simulink model "Missile_Aerodynamics"  (R2018a)
settings: Solver=ode4  StartTime=0.0  StopTime=5  FixedStep=Step_Size  RelTol=1e-3  EnableMultiTasking=on
InitFcn:
  | clc ;
  | clear all ;
  | close all ;
  | Missile_Data ;
  | Sim_Parameters ;
undefined symbols (not defined in the file): ALT, D, K_A, K_DC, K_p, K_phi, K_R, Mass, Omega_i, S, SOS_Table, Tbl_ALPHAT, Tbl_CL_ALPHAT, Tbl_CL_DEL_R, Tbl_CL_P, Tbl_CM_0, Tbl_CM_DEL_P, Tbl_CM_PHIT, Tbl_CM_Q, Tbl_CN_DEL_Y, Tbl_CN_PHIT, Tbl_CN_R, Tbl_CX_0, Tbl_CX_ALPHAT, Tbl_CX_DEL_EFF, Tbl_CY_DEL_Y, Tbl_CY_PHIT, Tbl_CZ_0, Tbl_CZ_DEL_P, Tbl_CZ_PHIT, Tbl_MACH, UNIT_GRAV, Wn_Act, XCG, XREF, Zeta_Act
libraries: simulink_extras x8, aerolibtransform2 x4, aerolibconvert2 x3, aerolibasang x3, UAS_Model_library x2, shared6dof x1
settings Model: Creator=e803534  LastModifiedBy=s293701
settings OptimizationCC: LifeSpan=inf
settings DebuggingCC: UnconnectedInputMsg=none  UnconnectedOutputMsg=none  UnconnectedLineMsg=none  LibraryContextMissingDiagnostic=warning  SFUnexpectedBacktrackingDiag=warning  SFNoUnconditionalDefaultTransitionDiag=warning
settings CodeAppCC: StateflowObjectComments=on
settings GRTTargetCC: TargetLangStandard=C89/C90 (ANSI)  GeneratePreprocessorConditionals=Disable all
settings ConfigComp: CovMetricSettings=dw  CovHtmlReporting=on  CovSaveCumulativeToWorkspaceVar=on  CovSaveSingleToWorkspaceVar=on  CovExternalEMLEnable=off

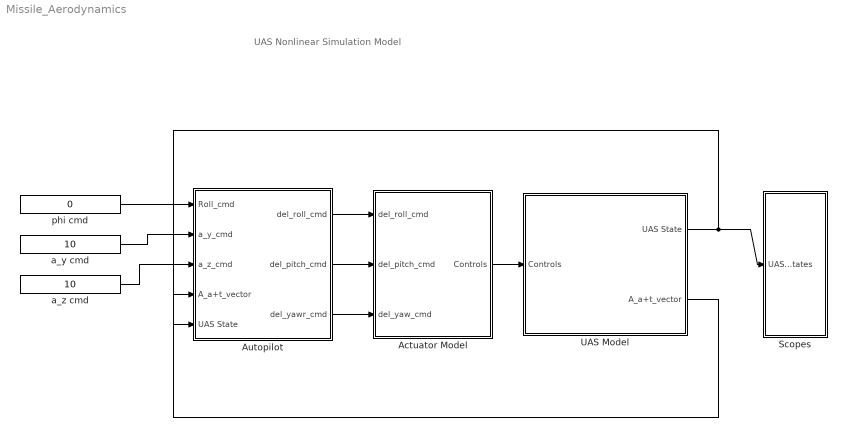
== system Missile_Aerodynamics ==
  note: UAS Nonlinear Simulation Model
  Actuator Model : Subsystem
  "Autopilot " : Subsystem
  Scopes : Subsystem
  UAS Model : Subsystem
  a_y cmd : Constant  Value=10
  a_z cmd : Constant  Value=10
  phi cmd : Constant  Value=0
  wires:
  "Autopilot "/2(del_pitch_cmd) -> Actuator Model/2(del_pitch_cmd)
  "Autopilot "/1(del_roll_cmd) -> Actuator Model/1(del_roll_cmd)
  "Autopilot "/3(del_yawr_cmd) -> Actuator Model/3(del_yaw_cmd)
  UAS Model/1(UAS State) -> "Autopilot "/5(UAS State), Scopes/1(UAS States)
  a_z cmd/1 -> "Autopilot "/3(a_z_cmd)
  phi cmd/1 -> "Autopilot "/1(Roll_cmd)
  a_y cmd/1 -> "Autopilot "/2(a_y_cmd)
  UAS Model/2(A_a+t_vector) -> "Autopilot "/4(A_a+t_vector)
  Actuator Model/1(Controls) -> UAS Model/1(Controls)

== system Missile_Aerodynamics/Actuator Model ==
  note: Actuator Models
  del_roll_cmd : Inport
  del_pitch_cmd : Inport  Port=2
  del_yaw_cmd : Inport  Port=3
  Display : Display
  Display1 : Display
  Display2 : Display
  Mux : Mux  Inputs=3
  Radians to Degrees : simulink_extras/Transformations/Radians to Degrees
  Saturation : Saturate  UpperLimit=10  LowerLimit=-10
  Saturation1 : Saturate  UpperLimit=10  LowerLimit=-10
  Saturation2 : Saturate  UpperLimit=10  LowerLimit=-10
  Scope1 : Scope
  Transfer Fcn : TransferFcn  Numerator=[Wn_Act^2]  Denominator=[1 2*Zeta_Act*Wn_Act Wn_Act^2]
  Transfer Fcn1 : TransferFcn  Numerator=[Wn_Act^2]  Denominator=[1 2*Zeta_Act*Wn_Act Wn_Act^2]
  Transfer Fcn2 : TransferFcn  Numerator=[Wn_Act^2]  Denominator=[1 2*Zeta_Act*Wn_Act Wn_Act^2]
  Controls : Outport
  wires:
  del_roll_cmd/1 -> Transfer Fcn/1
  Mux/1 -> Radians to Degrees/1, Controls/1
  del_yaw_cmd/1 -> Transfer Fcn2/1
  del_pitch_cmd/1 -> Transfer Fcn1/1
  Transfer Fcn/1 -> Saturation/1, Display/1
  Transfer Fcn1/1 -> Display1/1, Saturation1/1
  Transfer Fcn2/1 -> Saturation2/1, Display2/1
  Saturation/1 -> Mux/1
  Saturation2/1 -> Mux/3
  Saturation1/1 -> Mux/2
  Radians to Degrees/1 -> Scope1/1

== system Missile_Aerodynamics/Autopilot  ==
  note: Autopilot
  Roll_cmd : Inport
  a_y_cmd : Inport  Port=2
  a_z_cmd : Inport  Port=3
  A_a+t_vector : Inport  Port=4
  UAS State : Inport  Port=5
  Mux : Mux  Inputs=3
  Pitch Control : Subsystem  AncestorBlock=UAS_Model_library/Autopilot/Pitch Control
  Roll Control : Subsystem  AncestorBlock=UAS_Model_library/Autopilot/Roll Control
  Scope : Scope
  "Yaw Control " : Subsystem  AncestorBlock=UAS_Model_library/Autopilot/Yaw SAS
  del_roll_cmd : Outport
  del_pitch_cmd : Outport  Port=2
  del_yawr_cmd : Outport  Port=3
  wires:
  UAS State/1 -> Pitch Control/2(UAS_State), Roll Control/2(UAS_State), "Yaw Control "/1(UAS_State)
  a_z_cmd/1 -> Pitch Control/1(a_z_cmd)
  Pitch Control/1(del_p_cmd) -> Mux/2, del_pitch_cmd/1
  Roll_cmd/1 -> Roll Control/1(Roll_cmd)
  Roll Control/1(del_r_cmd) -> Mux/1, del_roll_cmd/1
  a_y_cmd/1 -> "Yaw Control "/2("a_y_cmd ")
  "Yaw Control "/1(del_r_cmd) -> Mux/3, del_yawr_cmd/1
  A_a+t_vector/1 -> Pitch Control/3(A_a+t_vector), "Yaw Control "/3(A_a+t_vector)
  Mux/1 -> Scope/1

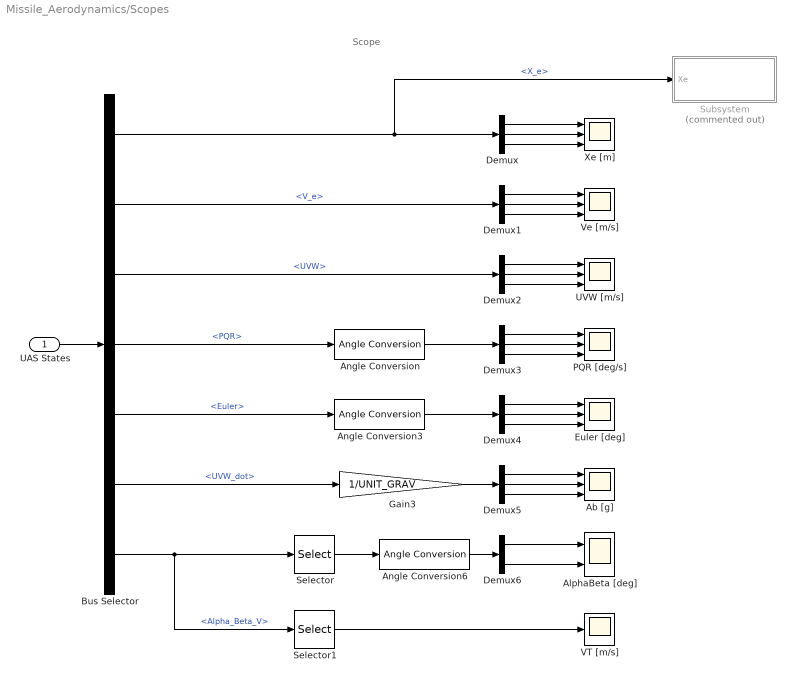
== system Missile_Aerodynamics/Scopes ==
  note: Scope
  UAS States : Inport
  Ab [g] : Scope  NumInputPorts=3
  AlphaBeta [deg] : Scope  NumInputPorts=2
  Angle Conversion : aerolibconvert2/Angle Conversion  IU=rad  OU=deg
  Angle Conversion3 : aerolibconvert2/Angle Conversion  IU=rad  OU=deg
  Angle Conversion6 : aerolibconvert2/Angle Conversion  IU=rad  OU=deg
  Bus Selector : BusSelector  OutputSignals=X_e,V_e,UVW,PQR,Euler,UVW_dot,Alpha_Beta_V
  Demux{,1..5} (6 alike) : Demux  Outputs=3
  Demux6 : Demux  Outputs=2
  Euler [deg] : Scope  NumInputPorts=3
  Gain3 : Gain  Gain=1/UNIT_GRAV
  PQR [deg/s] : Scope  NumInputPorts=3
  Selector : Selector  InputPortWidth=3  IndexOptions=Index vector (dialog)  Indices=[1 2]  OutputSizes=1
  Selector1 : Selector  InputPortWidth=3  IndexOptions=Index vector (dialog)  Indices=[3]  OutputSizes=1
  Subsystem : Subsystem  Commented=on
  UVW [m/s] : Scope  NumInputPorts=3
  VT [m/s] : Scope
  Ve [m/s] : Scope  NumInputPorts=3
  Xe [m] : Scope  NumInputPorts=3
  wires:
  UAS States/1 -> Bus Selector/1
  Bus Selector/1 -> Subsystem/1(Xe), Demux/1  "<X_e>"
  Bus Selector/2 -> Demux1/1  "<V_e>"
  Bus Selector/3 -> Demux2/1  "<UVW>"
  Bus Selector/4 -> Angle Conversion/1  "<PQR>"
  Bus Selector/5 -> Angle Conversion3/1  "<Euler>"
  Bus Selector/6 -> Gain3/1  "<UVW_dot>"
  Angle Conversion3/1 -> Demux4/1
  Angle Conversion/1 -> Demux3/1
  Selector1/1 -> VT [m/s]/1
  Gain3/1 -> Demux5/1
  Demux/1 -> Xe [m]/1
  Demux/2 -> Xe [m]/2
  Demux/3 -> Xe [m]/3
  Demux1/1 -> Ve [m/s]/1
  Demux1/2 -> Ve [m/s]/2
  Demux1/3 -> Ve [m/s]/3
  Demux2/1 -> UVW [m/s]/1
  Demux2/2 -> UVW [m/s]/2
  Demux2/3 -> UVW [m/s]/3
  Demux3/1 -> PQR [deg/s]/1
  Demux3/2 -> PQR [deg/s]/2
  Demux3/3 -> PQR [deg/s]/3
  Demux4/1 -> Euler [deg]/1
  Demux4/2 -> Euler [deg]/2
  Demux4/3 -> Euler [deg]/3
  Demux5/1 -> Ab [g]/1
  Demux5/2 -> Ab [g]/2
  Demux5/3 -> Ab [g]/3
  Demux6/2 -> AlphaBeta [deg]/2
  Demux6/1 -> AlphaBeta [deg]/1
  Angle Conversion6/1 -> Demux6/1
  Bus Selector/7 -> Selector1/1, Selector/1  "<Alpha_Beta_V>"
  Selector/1 -> Angle Conversion6/1

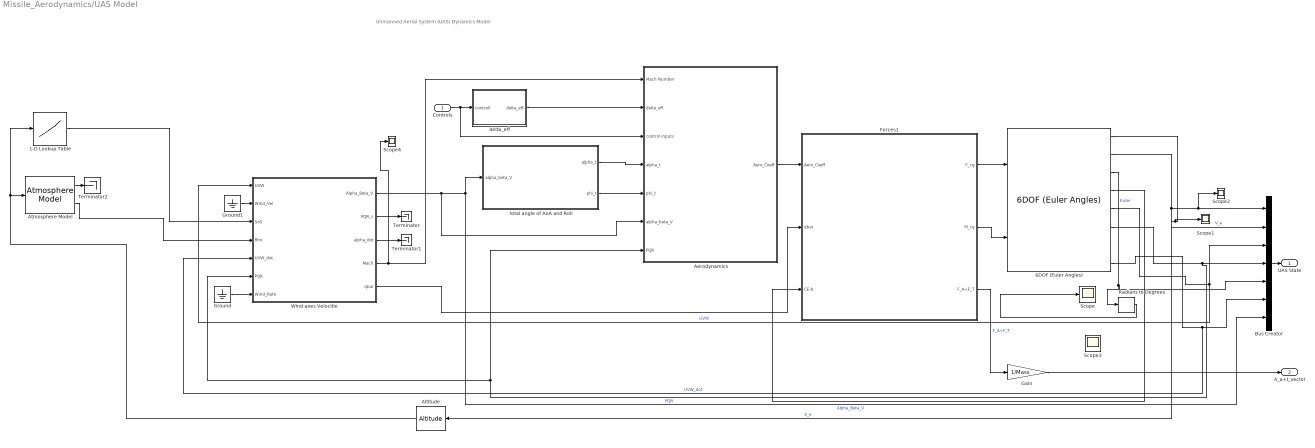
== system Missile_Aerodynamics/UAS Model ==
  note: Unmanned Aerial System (UAS) Dynamics Model
  Controls : Inport
  1-D Lookup Table : Lookup_n-D  NumberOfTableDimensions=1  BreakpointsForDimension1=ALT  Table=SOS_Table  InternalRulePriority=Speed  RndMeth=Simplest  InputSameDT=on
  6DOF (Euler Angles) : shared6dof/6DOF (Euler Angles)  units=Metric (MKS)  mtype=Fixed  rep=Euler Angles  xme_0=Init_Pos  Vm_0=Init_Vel  eul_0=Init_Euler  pm_0=Init_Rate  mass_0=Mass  mass_e=0.5  mass_f=2.0  inertia=I_TENSOR  inertia_e=eye(3)  inertia_f=2*eye(3)  k_quat=1.0  vre_flag=on  abi_flag=off  aMode=0
      settings: SourceProductBaseCode=AE
  Aerodynamics : Subsystem
  Altitude : UAS_Model_library/Equations of Motion/Altitude
  Atmosphere Model : UAS_Model_library/Envrionment/Atmosphere Model
  Bus Creator : BusCreator  Inputs=7
  Forces1 : Subsystem
  Gain : Gain  Gain=1/Mass
  Ground : Ground
  Ground1 : Ground
  Radians to Degrees : simulink_extras/Transformations/Radians to Degrees
  Scope{,1..4} (5 alike) : Scope
  Terminator : Terminator
  Terminator1 : Terminator
  Terminator2 : Terminator
  Wind-axes Velocitie : Subsystem  AncestorBlock=UAS_Model_library/External Forces/Aerodynamics/Wind-axes Velocitie
  delta_eff : Subsystem
  total angle of AoA and Roll : Subsystem
  UAS State : Outport
  A_a+t_vector : Outport  Port=2
  wires:
  Wind-axes Velocitie/1(Alpha_Beta_V) -> Aerodynamics/6(alpha_beta_V), total angle of AoA and Roll/1(alpha_beta_V), Bus Creator/7  "Alpha_Beta_V"
  total angle of AoA and Roll/2(phi_t) -> Aerodynamics/5(phi_t)
  delta_eff/1(delta_eff) -> Aerodynamics/2(delta_eff)
  Atmosphere Model/2 -> Wind-axes Velocitie/4(Rho)
  6DOF (Euler Angles)/8 -> Bus Creator/6, Wind-axes Velocitie/5(UVW_dot)  "UVW_dot"
  total angle of AoA and Roll/1(alpha_t) -> Aerodynamics/4(alpha_t)
  Wind-axes Velocitie/4(Mach) -> Scope4/1, Aerodynamics/1(Mach Number)
  6DOF (Euler Angles)/5 -> Wind-axes Velocitie/1(UVW), Bus Creator/3  "UVW"
  Ground1/1 -> Wind-axes Velocitie/2(Wind_Vel)
  Forces1/1(F_cg) -> 6DOF (Euler Angles)/1
  Aerodynamics/1(Aero_Coeff) -> Forces1/1(Aero_Coeff)
  Forces1/2(M_cg) -> 6DOF (Euler Angles)/2
  6DOF (Euler Angles)/6 -> Wind-axes Velocitie/6(PQR), Aerodynamics/7(PQR), Bus Creator/4  "PQR"
  Controls/1 -> Aerodynamics/3(control inputs), delta_eff/1(controll)
  Wind-axes Velocitie/5(qbar) -> Forces1/2(qbar)
  Ground/1 -> Wind-axes Velocitie/7(Wind_Rate)
  Bus Creator/1 -> UAS State/1
  6DOF (Euler Angles)/2 -> Altitude/1, Scope2/1, Bus Creator/1  "X_e"
  6DOF (Euler Angles)/1 -> Bus Creator/2, Scope1/1  "V_e"
  6DOF (Euler Angles)/3 -> Radians to Degrees/1, Bus Creator/5  "Euler"
  Forces1/3(F_A+F_T) -> Gain/1  "F_A+F_T"
  Wind-axes Velocitie/2(PQR_s) -> Terminator/1
  Wind-axes Velocitie/3(alpha_dot) -> Terminator1/1
  6DOF (Euler Angles)/4 -> Forces1/3(CE-b)
  Altitude/1 -> 1-D Lookup Table/1, Atmosphere Model/1
  Radians to Degrees/1 -> Scope/1
  Gain/1 -> A_a+t_vector/1
  Atmosphere Model/1 -> Terminator2/1
  1-D Lookup Table/1 -> Wind-axes Velocitie/3(SoS)

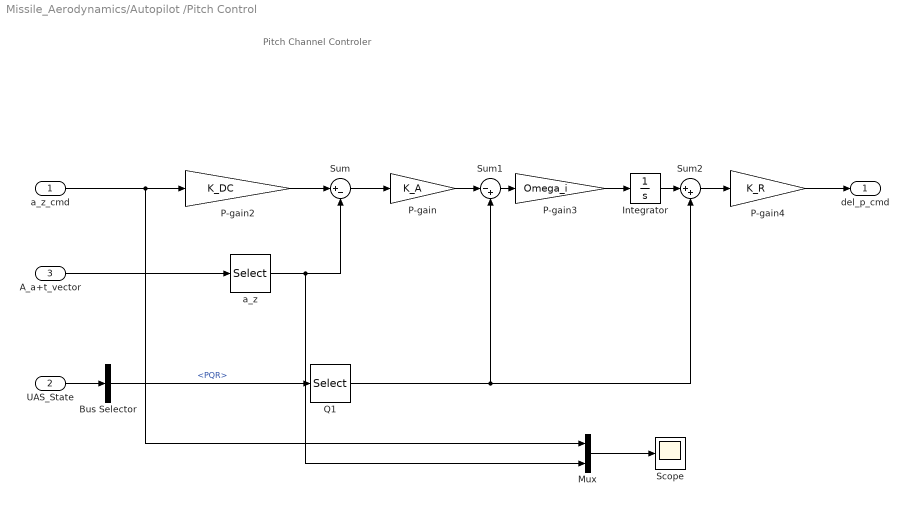
== system Missile_Aerodynamics/Autopilot /Pitch Control ==
  note: Pitch Channel Controler
  a_z_cmd : Inport
  UAS_State : Inport  Port=2
  A_a+t_vector : Inport  Port=3
  Bus Selector : BusSelector  OutputSignals=PQR
  Integrator : Integrator
  Mux : Mux  Inputs=2
  P-gain : Gain  Gain=K_A
  P-gain2 : Gain  Gain=K_DC
  P-gain3 : Gain  Gain=Omega_i
  P-gain4 : Gain  Gain=K_R
  Q1 : Selector  InputPortWidth=3  IndexOptions=Index vector (dialog)  Indices=[2]  OutputSizes=1
  Scope : Scope
  Sum : Sum  Inputs=|+-
  Sum1 : Sum  Inputs=|-+
  Sum2 : Sum  Inputs=|++
  a_z : Selector  InputPortWidth=3  IndexOptions=Index vector (dialog)  Indices=[3]  OutputSizes=1
  del_p_cmd : Outport
  wires:
  UAS_State/1 -> Bus Selector/1
  Bus Selector/1 -> Q1/1  "<PQR>"
  Sum2/1 -> P-gain4/1
  Sum1/1 -> P-gain3/1
  Q1/1 -> Sum2/2, Sum1/2
  P-gain/1 -> Sum1/1
  Sum/1 -> P-gain/1
  a_z_cmd/1 -> Mux/1, P-gain2/1
  P-gain2/1 -> Sum/1
  P-gain3/1 -> Integrator/1
  Integrator/1 -> Sum2/1
  P-gain4/1 -> del_p_cmd/1
  a_z/1 -> Mux/2, Sum/2
  A_a+t_vector/1 -> a_z/1
  Mux/1 -> Scope/1

== system Missile_Aerodynamics/Autopilot /Roll Control ==
  note: Roll Control
  Roll_cmd : Inport
  UAS_State : Inport  Port=2
  Bus Selector : BusSelector  OutputSignals=Euler,PQR
  P : Selector  InputPortWidth=3  IndexOptions=Index vector (dialog)  Indices=[1]  OutputSizes=1
  P-gain2 : Gain  Gain=K_phi
  P-gain3 : Gain  Gain=K_p
  PHI : Selector  InputPortWidth=3  IndexOptions=Index vector (dialog)  Indices=[1]  OutputSizes=1
  Sum : Sum  Inputs=|+-
  Sum2 : Sum  Inputs=|+-
  del_r_cmd : Outport
  wires:
  Bus Selector/2 -> P/1  "<PQR>"
  Bus Selector/1 -> PHI/1  "<Euler>"
  UAS_State/1 -> Bus Selector/1
  PHI/1 -> Sum/2
  Roll_cmd/1 -> Sum/1
  P-gain2/1 -> Sum2/1
  P/1 -> Sum2/2
  Sum2/1 -> P-gain3/1
  Sum/1 -> P-gain2/1
  P-gain3/1 -> del_r_cmd/1

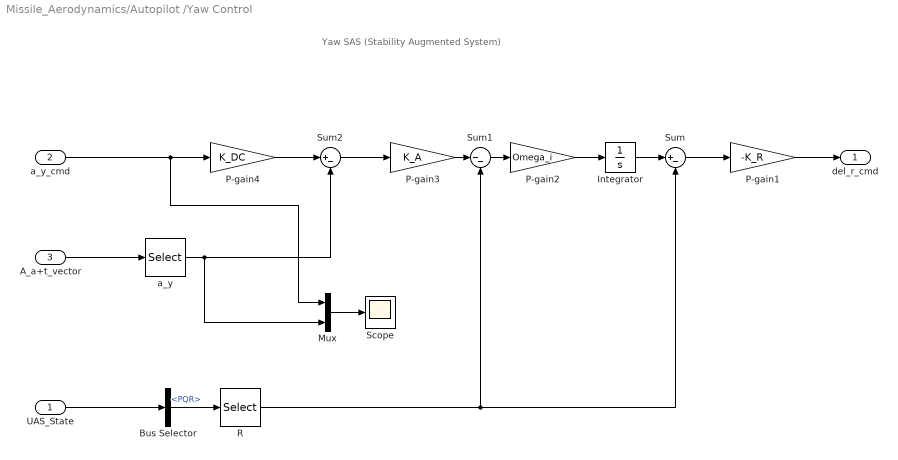
== system Missile_Aerodynamics/Autopilot /Yaw Control  ==
  note: Yaw SAS (Stability Augmented System)
  UAS_State : Inport
  "a_y_cmd " : Inport  Port=2
  A_a+t_vector : Inport  Port=3
  Bus Selector : BusSelector  OutputSignals=PQR
  Integrator : Integrator
  Mux : Mux  Inputs=2
  P-gain1 : Gain  Gain=-K_R
  P-gain2 : Gain  Gain=Omega_i
  P-gain3 : Gain  Gain=K_A
  P-gain4 : Gain  Gain=K_DC
  R : Selector  InputPortWidth=3  IndexOptions=Index vector (dialog)  Indices=[3]  OutputSizes=1
  Scope : Scope
  Sum : Sum  Inputs=|+-
  Sum1 : Sum  Inputs=|--
  Sum2 : Sum  Inputs=|+-
  a_y : Selector  InputPortWidth=3  IndexOptions=Index vector (dialog)  Indices=[2]  OutputSizes=1
  del_r_cmd : Outport
  wires:
  P-gain1/1 -> del_r_cmd/1
  P-gain2/1 -> Integrator/1
  Sum/1 -> P-gain1/1
  Integrator/1 -> Sum/1
  Sum1/1 -> P-gain2/1
  P-gain3/1 -> Sum1/1
  Sum2/1 -> P-gain3/1
  Bus Selector/1 -> R/1  "<PQR>"
  P-gain4/1 -> Sum2/1
  R/1 -> Sum1/2, Sum/2
  "a_y_cmd "/1 -> Mux/1, P-gain4/1
  UAS_State/1 -> Bus Selector/1
  A_a+t_vector/1 -> a_y/1
  a_y/1 -> Mux/2, Sum2/2
  Mux/1 -> Scope/1

== system Missile_Aerodynamics/Scopes/Subsystem ==
  Xe : Inport
  Constant : Constant
  Constant1 : Constant  Value=0
  Selector : Selector  InputPortWidth=3  IndexOptions=Index vector (dialog)  Indices=[3]  OutputSizes=1
  Stop Simulation : Stop
  Switch : Switch  Criteria=u2 > Threshold
  wires:
  Xe/1 -> Selector/1
  Selector/1 -> Switch/2
  Constant/1 -> Switch/1
  Constant1/1 -> Switch/3
  Switch/1 -> Stop Simulation/1

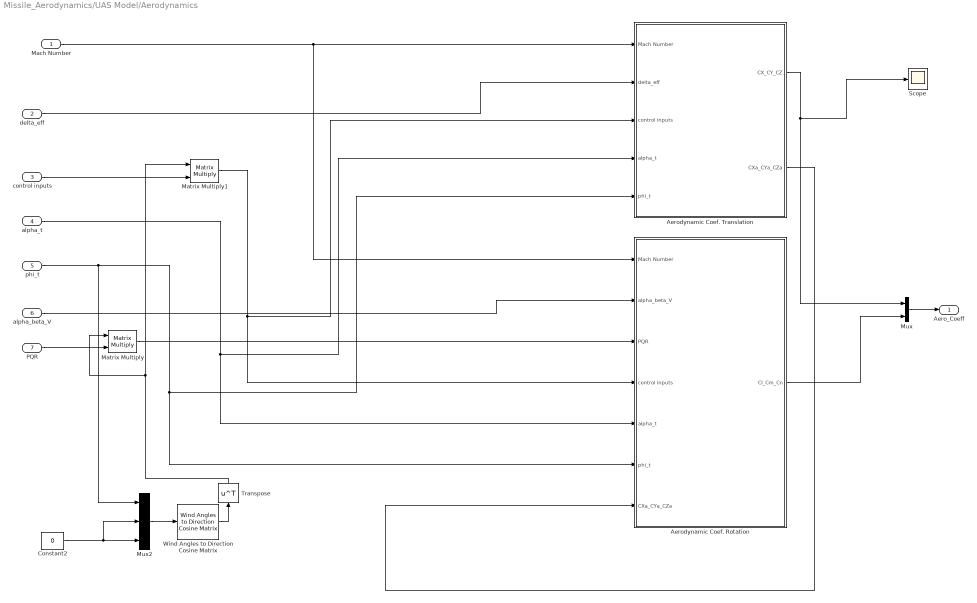
== system Missile_Aerodynamics/UAS Model/Aerodynamics ==
  Mach Number : Inport
  delta_eff : Inport  Port=2
  control inputs : Inport  Port=3
  alpha_t : Inport  Port=4
  phi_t : Inport  Port=5
  alpha_beta_V : Inport  Port=6
  PQR : Inport  Port=7
  Aerodynamic Coef. Rotation : Subsystem
  Aerodynamic Coef. Translation : Subsystem
  Constant2 : Constant  Value=0
  Matrix Multiply : Product  Multiplication=Matrix(*)
  Matrix Multiply1 : Product  Multiplication=Matrix(*)
  Mux : Mux  Inputs=2
  Mux2 : Mux  Inputs=3
  Scope : Scope
  Transpose : Math  Operator=transpose  SaturateOnIntegerOverflow=on
  Wind Angles to Direction Cosine Matrix : aerolibtransform2/Wind Angles to  Direction Cosine Matrix
      settings: SourceProductName=Aerospace Blockset  SourceProductBaseCode=AE
  Aero_Coeff : Outport
  wires:
  Aerodynamic Coef. Translation/2(CXa_CYa_CZa) -> Aerodynamic Coef. Rotation/7(CXa_CYa_CZa)
  Mach Number/1 -> Aerodynamic Coef. Rotation/1(Mach Number), Aerodynamic Coef. Translation/1(Mach Number)
  delta_eff/1 -> Aerodynamic Coef. Translation/2(delta_eff)
  Matrix Multiply1/1 -> Aerodynamic Coef. Rotation/4(control inputs), Aerodynamic Coef. Translation/3(control inputs)
  alpha_beta_V/1 -> Aerodynamic Coef. Rotation/2(alpha_beta_V)
  Matrix Multiply/1 -> Aerodynamic Coef. Rotation/3(PQR)
  Aerodynamic Coef. Translation/1(CX_CY_CZ) -> Scope/1, Mux/1
  Aerodynamic Coef. Rotation/1(Cl_Cm_Cn) -> Mux/2
  Mux/1 -> Aero_Coeff/1
  alpha_t/1 -> Aerodynamic Coef. Rotation/5(alpha_t), Aerodynamic Coef. Translation/4(alpha_t)
  phi_t/1 -> Mux2/1, Aerodynamic Coef. Translation/5(phi_t), Aerodynamic Coef. Rotation/6(phi_t)
  Mux2/1 -> Wind Angles to Direction Cosine Matrix/1
  Constant2/1 -> Mux2/2, Mux2/3
  control inputs/1 -> Matrix Multiply1/2
  Wind Angles to Direction Cosine Matrix/1 -> Transpose/1
  PQR/1 -> Matrix Multiply/2
  Transpose/1 -> Matrix Multiply/1, Matrix Multiply1/1

== system Missile_Aerodynamics/UAS Model/Forces1 ==
  Aero_Coeff : Inport
  qbar : Inport  Port=2
  CE-b : Inport  Port=3
  Aerodynamic Force & Moment : Subsystem  AncestorBlock=UAS_Model_library/External Forces/Aerodynamics/Aerodynamic Force & Moment
  Propulsive Force & Moment : Subsystem  AncestorBlock=UAS_Model_library/External Forces/Propulsive/Propulsive Force & Moment
  Sum of Aerodynamic and Propulsion Forces : Sum
  Total Force & Moment : Subsystem  AncestorBlock=UAS_Model_library/External Forces/Total Force & Moment
  F_cg : Outport
  M_cg : Outport  Port=2
  F_A+F_T : Outport  Port=3
  wires:
  Total Force & Moment/2(M_cg) -> M_cg/1
  Aerodynamic Force & Moment/2(M_aero) -> Total Force & Moment/2(M_aero)
  Propulsive Force & Moment/2(M_prop) -> Total Force & Moment/4(M_prop)
  Total Force & Moment/1(F_cg) -> F_cg/1
  Aerodynamic Force & Moment/1(F_aero) -> Sum of Aerodynamic and Propulsion Forces/1, Total Force & Moment/1(F_aero)
  Propulsive Force & Moment/1(F_prop) -> Sum of Aerodynamic and Propulsion Forces/2, Total Force & Moment/3(F_prop)
  qbar/1 -> Aerodynamic Force & Moment/2(qbar)
  Aero_Coeff/1 -> Aerodynamic Force & Moment/1(Aero_Coeff)
  Sum of Aerodynamic and Propulsion Forces/1 -> F_A+F_T/1
  CE-b/1 -> Total Force & Moment/5("cE-B ")

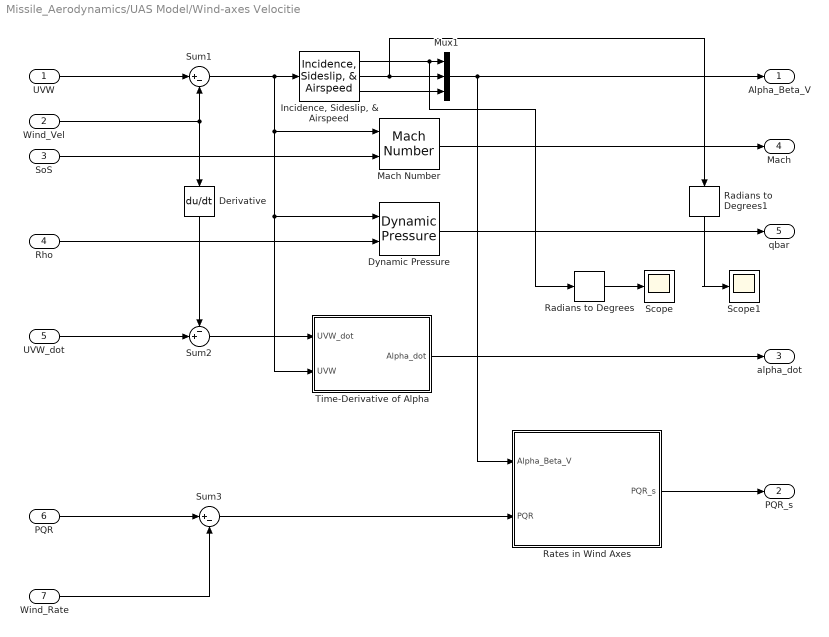
== system Missile_Aerodynamics/UAS Model/Wind-axes Velocitie ==
  UVW : Inport
  Wind_Vel : Inport  Port=2
  SoS : Inport  Port=3
  Rho : Inport  Port=4
  UVW_dot : Inport  Port=5
  PQR : Inport  Port=6
  Wind_Rate : Inport  Port=7
  Derivative : Derivative
  Dynamic Pressure : aerolibasang/Dynamic Pressure
  "Incidence, Sideslip, & Airspeed" : aerolibasang/Incidence, Sideslip, & Airspeed
      settings: SourceProductName=Aerospace Blockset
  Mach Number : aerolibasang/Mach Number
      settings: SourceProductName=Aerospace Blockset  SourceProductBaseCode=AE
  Mux1 : Mux  Inputs=3
  Radians to Degrees : simulink_extras/Transformations/Radians to Degrees
  Radians to Degrees1 : simulink_extras/Transformations/Radians to Degrees
  Rates in Wind Axes : Subsystem
  Scope : Scope
  Scope1 : Scope
  Sum1 : Sum  Inputs=|+-  SaturateOnIntegerOverflow=on  InputSameDT=on  OutDataTypeStr=Inherit: Same as first input
  Sum2 : Sum  Inputs=-+|  SaturateOnIntegerOverflow=on  InputSameDT=on  OutDataTypeStr=Inherit: Same as first input
  Sum3 : Sum  Inputs=|+-  SaturateOnIntegerOverflow=on  InputSameDT=on  OutDataTypeStr=Inherit: Same as first input
  Time-Derivative of Alpha : Subsystem
  Alpha_Beta_V : Outport
  PQR_s : Outport  Port=2
  alpha_dot : Outport  Port=3
  Mach : Outport  Port=4
  qbar : Outport  Port=5
  wires:
  Wind_Rate/1 -> Sum3/2
  PQR/1 -> Sum3/1
  Sum3/1 -> Rates in Wind Axes/2(PQR)
  Rates in Wind Axes/1(PQR_s) -> PQR_s/1
  "Incidence, Sideslip, & Airspeed"/3 -> Mux1/3
  "Incidence, Sideslip, & Airspeed"/2 -> Radians to Degrees1/1, Mux1/2
  "Incidence, Sideslip, & Airspeed"/1 -> Radians to Degrees/1, Mux1/1
  Sum1/1 -> "Incidence, Sideslip, & Airspeed"/1, Mach Number/1, Dynamic Pressure/1, Time-Derivative of Alpha/2(UVW)
  Mux1/1 -> Alpha_Beta_V/1, Rates in Wind Axes/1(Alpha_Beta_V)
  UVW/1 -> Sum1/1
  Wind_Vel/1 -> Derivative/1, Sum1/2
  Mach Number/1 -> Mach/1
  SoS/1 -> Mach Number/2
  Rho/1 -> Dynamic Pressure/2
  Dynamic Pressure/1 -> qbar/1
  Time-Derivative of Alpha/1(Alpha_dot) -> alpha_dot/1
  UVW_dot/1 -> Sum2/2
  Sum2/1 -> Time-Derivative of Alpha/1(UVW_dot)
  Derivative/1 -> Sum2/1
  Radians to Degrees/1 -> Scope/1
  Radians to Degrees1/1 -> Scope1/1

== system Missile_Aerodynamics/UAS Model/delta_eff ==
  controll : Inport
  Abs : Abs
  Abs1 : Abs
  Constant : Constant  Value=2
  Divide : Product  Inputs=*/  SaturateOnIntegerOverflow=on  RndMeth=Zero
  Selector : Selector  InputPortWidth=3  IndexOptions=Index vector (dialog)  Indices=[3]  OutputSizes=1
  Selector1 : Selector  InputPortWidth=3  IndexOptions=Index vector (dialog)  Indices=[2]  OutputSizes=1
  Sum : Sum  Inputs=|++
  delta_eff : Outport
  wires:
  Selector1/1 -> Abs1/1
  Sum/1 -> Divide/1
  Constant/1 -> Divide/2
  Divide/1 -> delta_eff/1
  controll/1 -> Selector/1, Selector1/1
  Selector/1 -> Abs/1
  Abs/1 -> Sum/1
  Abs1/1 -> Sum/2

== system Missile_Aerodynamics/UAS Model/total angle of AoA and Roll ==
  alpha_beta_V : Inport
  Asin : Trigonometry  Operator=acos
  Atan2 : Trigonometry  Operator=atan2
  Cos : Trigonometry  Operator=cos
  Cos1 : Trigonometry  Operator=cos
  Multiply : Product
  Selector : Selector  InputPortWidth=3  IndexOptions=Index vector (dialog)  Indices=[1]  OutputSizes=1
  Selector1 : Selector  InputPortWidth=3  IndexOptions=Index vector (dialog)  Indices=[2]  OutputSizes=1
  Sin : Trigonometry
  Tan : Trigonometry  Operator=tan
  alpha_t : Outport
  phi_t : Outport  Port=2
  wires:
  Sin/1 -> Atan2/2
  Tan/1 -> Atan2/1
  Selector/1 -> Sin/1, Cos/1
  Selector1/1 -> Tan/1, Cos1/1
  Cos1/1 -> Multiply/2
  Multiply/1 -> Asin/1
  Cos/1 -> Multiply/1
  Atan2/1 -> phi_t/1
  Asin/1 -> alpha_t/1
  alpha_beta_V/1 -> Selector1/1, Selector/1

== system Missile_Aerodynamics/UAS Model/Aerodynamics/Aerodynamic Coef. Rotation ==
  Mach Number : Inport
  alpha_beta_V : Inport  Port=2
  PQR : Inport  Port=3
  control inputs : Inport  Port=4
  alpha_t : Inport  Port=5
  phi_t : Inport  Port=6
  CXa_CYa_CZa : Inport  Port=7
  Constant2 : Constant  Value=0
  Display1 : Display
  Matrix Multiply : Product  Multiplication=Matrix(*)
  Mux : Mux  Inputs=3
  Mux2 : Mux  Inputs=3
  Subsystem Aero. Coef. Rotation : Subsystem
  Wind Angles to Direction Cosine Matrix : aerolibtransform2/Wind Angles to  Direction Cosine Matrix
      settings: SourceProductName=Aerospace Blockset  SourceProductBaseCode=AE
  Cl_Cm_Cn : Outport
  wires:
  Mux/1 -> Matrix Multiply/2
  Matrix Multiply/1 -> Cl_Cm_Cn/1
  Mach Number/1 -> Subsystem Aero. Coef. Rotation/1(Mach Number)
  alpha_beta_V/1 -> Subsystem Aero. Coef. Rotation/4(alpha_beta_V)
  PQR/1 -> Subsystem Aero. Coef. Rotation/5(PQR)
  control inputs/1 -> Subsystem Aero. Coef. Rotation/6(control)
  alpha_t/1 -> Subsystem Aero. Coef. Rotation/2(alpha_t)
  phi_t/1 -> Mux2/1, Subsystem Aero. Coef. Rotation/3(phi_t)
  CXa_CYa_CZa/1 -> Subsystem Aero. Coef. Rotation/7(C_X_C_Y_CZ)
  Mux2/1 -> Wind Angles to Direction Cosine Matrix/1
  Constant2/1 -> Mux2/2, Mux2/3
  Wind Angles to Direction Cosine Matrix/1 -> Matrix Multiply/1
  Subsystem Aero. Coef. Rotation/1(C_L_A) -> Mux/1
  Subsystem Aero. Coef. Rotation/2(C_M_A) -> Display1/1, Mux/2
  Subsystem Aero. Coef. Rotation/3(C_N_A) -> Mux/3

== system Missile_Aerodynamics/UAS Model/Aerodynamics/Aerodynamic Coef. Translation ==
  Mach Number : Inport
  delta_eff : Inport  Port=2
  control inputs : Inport  Port=3
  alpha_t : Inport  Port=4
  phi_t : Inport  Port=5
  Constant2 : Constant  Value=0
  Matrix Multiply : Product  Multiplication=Matrix(*)
  Mux : Mux  Inputs=3
  Mux2 : Mux  Inputs=3
  Scope : Scope
  Subsystem Aero. Coef. Translation : Subsystem
  Transpose : Math  Commented=on  Operator=transpose  SaturateOnIntegerOverflow=on
  Wind Angles to Direction Cosine Matrix : aerolibtransform2/Wind Angles to  Direction Cosine Matrix
      settings: SourceProductName=Aerospace Blockset  SourceProductBaseCode=AE
  CX_CY_CZ : Outport
  CXa_CYa_CZa : Outport  Port=2
  wires:
  Mux/1 -> Matrix Multiply/2, CXa_CYa_CZa/1
  Matrix Multiply/1 -> CX_CY_CZ/1
  Mux2/1 -> Wind Angles to Direction Cosine Matrix/1
  phi_t/1 -> Mux2/1, Subsystem Aero. Coef. Translation/5(phi_t)
  Constant2/1 -> Mux2/2, Mux2/3
  Mach Number/1 -> Subsystem Aero. Coef. Translation/1(Mach number)
  control inputs/1 -> Subsystem Aero. Coef. Translation/4(control)
  alpha_t/1 -> Subsystem Aero. Coef. Translation/2(alpha_t)
  delta_eff/1 -> Subsystem Aero. Coef. Translation/3(delta_eff)
  Subsystem Aero. Coef. Translation/1(C_X_A) -> Scope/1, Mux/1
  Subsystem Aero. Coef. Translation/2(C_Y_A) -> Mux/2
  Subsystem Aero. Coef. Translation/3(C_Z_A) -> Mux/3
  Wind Angles to Direction Cosine Matrix/1 -> Matrix Multiply/1

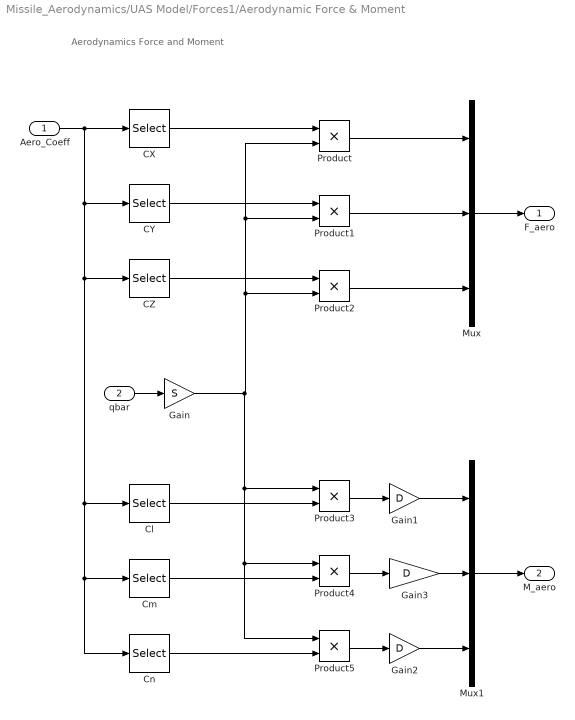
== system Missile_Aerodynamics/UAS Model/Forces1/Aerodynamic Force & Moment ==
  note: Aerodynamics Force and Moment
  Aero_Coeff : Inport
  qbar : Inport  Port=2
  CX : Selector  InputPortWidth=6  IndexOptions=Index vector (dialog)  Indices=[1]  OutputSizes=1
  CY : Selector  InputPortWidth=6  IndexOptions=Index vector (dialog)  Indices=[2]  OutputSizes=1
  CZ : Selector  InputPortWidth=6  IndexOptions=Index vector (dialog)  Indices=[3]  OutputSizes=1
  Cl : Selector  InputPortWidth=6  IndexOptions=Index vector (dialog)  Indices=[4]  OutputSizes=1
  Cm : Selector  InputPortWidth=6  IndexOptions=Index vector (dialog)  Indices=[5]  OutputSizes=1
  Cn : Selector  InputPortWidth=6  IndexOptions=Index vector (dialog)  Indices=[6]  OutputSizes=1
  Gain : Gain  Gain=S
  Gain1 : Gain  Gain=D
  Gain2 : Gain  Gain=D
  Gain3 : Gain  Gain=D
  Mux : Mux  Inputs=3
  Mux1 : Mux  Inputs=3
  Product{,1..5} (6 alike) : Product
  F_aero : Outport
  M_aero : Outport  Port=2
  wires:
  Gain3/1 -> Mux1/2
  Gain2/1 -> Mux1/3
  Gain1/1 -> Mux1/1
  Mux1/1 -> M_aero/1
  Product5/1 -> Gain2/1
  Product4/1 -> Gain3/1
  Product3/1 -> Gain1/1
  Cn/1 -> Product5/2
  Cm/1 -> Product4/2
  Cl/1 -> Product3/2
  Mux/1 -> F_aero/1
  Product2/1 -> Mux/3
  Product1/1 -> Mux/2
  Product/1 -> Mux/1
  CZ/1 -> Product2/1
  CY/1 -> Product1/1
  Gain/1 -> Product/2, Product1/2, Product2/2, Product3/1, Product4/1, Product5/1
  CX/1 -> Product/1
  qbar/1 -> Gain/1
  Aero_Coeff/1 -> CX/1, CY/1, CZ/1, Cm/1, Cn/1, Cl/1

== system Missile_Aerodynamics/UAS Model/Forces1/Propulsive Force & Moment ==
  note: Propulsive Force and Moment
  Constant : Constant  Value=0
  Constant1 : Constant  Value=0
  Mux : Mux  Inputs=3
  Mux1 : Mux  Inputs=3
  F_prop : Outport
  M_prop : Outport  Port=2
  wires:
  Mux/1 -> F_prop/1
  Constant/1 -> Mux/2, Mux1/1, Mux1/2, Mux1/3, Mux/3
  Mux1/1 -> M_prop/1
  Constant1/1 -> Mux/1

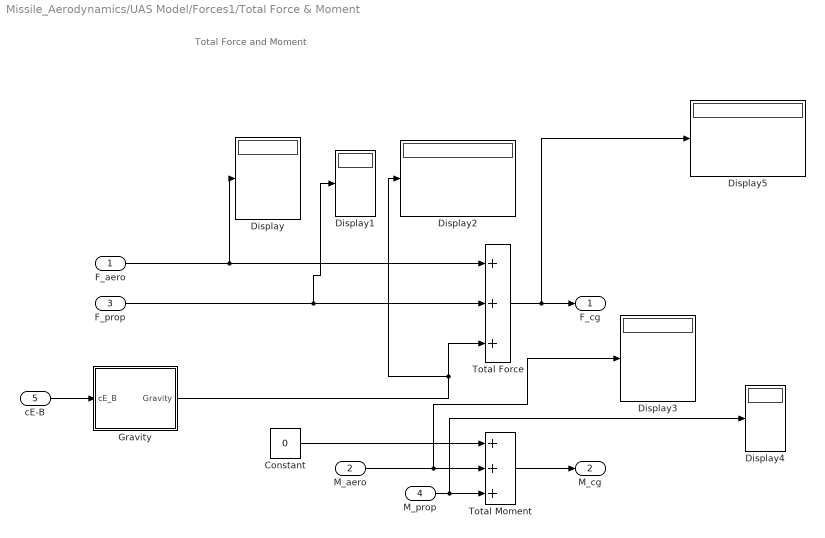
== system Missile_Aerodynamics/UAS Model/Forces1/Total Force & Moment ==
  note: Total Force and Moment
  F_aero : Inport  PortDimensions=3
  M_aero : Inport  Port=2  PortDimensions=3
  F_prop : Inport  Port=3  PortDimensions=3
  M_prop : Inport  Port=4  PortDimensions=3
  "cE-B " : Inport  Port=5
  Constant : Constant  Value=0
  Display{,1..5} (6 alike) : Display
  Gravity : Subsystem  AncestorBlock=UAS_Model_library/Envrionment/Gravity
  Total Force : Sum  Inputs=+++  SaturateOnIntegerOverflow=on  InputSameDT=on  OutDataTypeStr=Inherit: Same as first input
  Total Moment : Sum  Inputs=+++  SaturateOnIntegerOverflow=on  InputSameDT=on  OutDataTypeStr=Inherit: Same as first input
  F_cg : Outport
  M_cg : Outport  Port=2
  wires:
  Gravity/1(Gravity) -> Total Force/3, Display2/1
  Total Moment/1 -> M_cg/1
  M_prop/1 -> Display4/1, Total Moment/3
  F_prop/1 -> Display1/1, Total Force/2
  F_aero/1 -> Display/1, Total Force/1
  Constant/1 -> Total Moment/1
  M_aero/1 -> Display3/1, Total Moment/2
  "cE-B "/1 -> Gravity/1(cE_B)
  Total Force/1 -> Display5/1, F_cg/1

== system Missile_Aerodynamics/UAS Model/Wind-axes Velocitie/Rates in Wind Axes ==
  note: Rates in Wind Axes
  Alpha_Beta_V : Inport
  PQR : Inport  Port=2
  Alpha : Selector  InputPortWidth=3  IndexOptions=Index vector (dialog)  Indices=[1]  OutputSizes=1
  Beta_Ref : Constant  Value=0
  Direction Cosine Matrix Body to Wind : aerolibtransform2/Direction Cosine Matrix Body to Wind
      settings: SourceProductName=Aerospace Blockset  SourceProductBaseCode=AE
  Mux : Mux  Inputs=2
  transform to body axes : Product  Inputs=**  Multiplication=Matrix(*)  SaturateOnIntegerOverflow=on  InputSameDT=on  OutDataTypeStr=Inherit: Same as first input
  PQR_s : Outport
  wires:
  Beta_Ref/1 -> Mux/2
  Mux/1 -> Direction Cosine Matrix Body to Wind/1
  transform to body axes/1 -> PQR_s/1
  PQR/1 -> transform to body axes/2
  Direction Cosine Matrix Body to Wind/1 -> transform to body axes/1  "cB_W"
  Alpha/1 -> Mux/1
  Alpha_Beta_V/1 -> Alpha/1

== system Missile_Aerodynamics/UAS Model/Wind-axes Velocitie/Time-Derivative of Alpha ==
  note: Time Derivative of Alpha
  UVW_dot : Inport
  UVW : Inport  Port=2
  Add : Sum  Inputs=-+
  Add1 : Sum
  Demux2 : Demux  Outputs=3
  Demux3 : Demux  Outputs=3
  Divide : Product  Inputs=*/
  Math Function2 : Math  Operator=square  SaturateOnIntegerOverflow=on
  Math Function3 : Math  Operator=square  SaturateOnIntegerOverflow=on
  Product3 : Product
  Product4 : Product
  Terminator2 : Terminator
  Terminator3 : Terminator
  Alpha_dot : Outport
  wires:
  Divide/1 -> Alpha_dot/1
  Add1/1 -> Divide/2
  Math Function3/1 -> Add1/2
  Math Function2/1 -> Add1/1
  Add/1 -> Divide/1
  Product3/1 -> Add/1
  Product4/1 -> Add/2
  Demux3/1 -> Product4/2, Math Function2/1
  Demux2/3 -> Product4/1
  Demux3/3 -> Product3/2, Math Function3/1
  Demux3/2 -> Terminator3/1
  UVW/1 -> Demux3/1
  Demux2/1 -> Product3/1
  Demux2/2 -> Terminator2/1
  UVW_dot/1 -> Demux2/1

== system Missile_Aerodynamics/UAS Model/Aerodynamics/Aerodynamic Coef. Rotation/Subsystem Aero. Coef. Rotation ==
  Mach Number : Inport
  alpha_t : Inport  Port=2
  phi_t : Inport  Port=3
  alpha_beta_V : Inport  Port=4
  PQR : Inport  Port=5
  control : Inport  Port=6
  C_X_C_Y_CZ : Inport  Port=7
  "Subsystem C_L_A " : Subsystem
  "Subsystem C_M_A " : Subsystem
  Subsystem C_N_A : Subsystem
  C_L_A : Outport
  C_M_A : Outport  Port=2
  C_N_A : Outport  Port=3
  wires:
  "Subsystem C_M_A "/1(C_M_A) -> C_M_A/1
  "Subsystem C_L_A "/1(C_L_A) -> C_L_A/1
  Subsystem C_N_A/1(C_N_A) -> C_N_A/1
  Mach Number/1 -> "Subsystem C_L_A "/1(Mach Number), "Subsystem C_M_A "/1(Mach Number), Subsystem C_N_A/1(Mach Number)
  alpha_t/1 -> Subsystem C_N_A/2(alpha_t), "Subsystem C_M_A "/2(alpha_t), "Subsystem C_L_A "/2(alpha_t)
  phi_t/1 -> Subsystem C_N_A/3(phi_t), "Subsystem C_M_A "/3(phi_t), "Subsystem C_L_A "/3(phi_t)
  alpha_beta_V/1 -> "Subsystem C_L_A "/4(alpha_beta_V), "Subsystem C_M_A "/4(alpha_beta_V), Subsystem C_N_A/4(alpha_beta_V)
  PQR/1 -> "Subsystem C_M_A "/5(PQR), "Subsystem C_L_A "/5(PQR), Subsystem C_N_A/5(PQR)
  control/1 -> "Subsystem C_M_A "/6(control), "Subsystem C_L_A "/6(control), Subsystem C_N_A/6(control)
  C_X_C_Y_CZ/1 -> "Subsystem C_M_A "/7(C_X_C_Y_C_Z), Subsystem C_N_A/7(C_X_C_Y_C_Z)

== system Missile_Aerodynamics/UAS Model/Aerodynamics/Aerodynamic Coef. Translation/Subsystem Aero. Coef. Translation ==
  Mach number : Inport
  alpha_t : Inport  Port=2
  delta_eff : Inport  Port=3
  control : Inport  Port=4
  phi_t : Inport  Port=5
  Subsystem C_X_A : Subsystem
  Subsystem C_Y_A : Subsystem
  Subsystem C_Z_A : Subsystem
  C_X_A : Outport
  C_Y_A : Outport  Port=2
  C_Z_A : Outport  Port=3
  wires:
  Subsystem C_X_A/1(C_X_A) -> C_X_A/1
  Subsystem C_Y_A/1(C_Y_A) -> C_Y_A/1
  Subsystem C_Z_A/1(C_Z_A) -> C_Z_A/1
  Mach number/1 -> Subsystem C_Z_A/1(Mach Number), Subsystem C_Y_A/1(Mach Number), Subsystem C_X_A/1(Mach Number)
  alpha_t/1 -> Subsystem C_Z_A/2(alpha_t), Subsystem C_Y_A/2(alpha_t), Subsystem C_X_A/2(alpha_t)
  delta_eff/1 -> Subsystem C_X_A/3(delta_eff)
  control/1 -> Subsystem C_Z_A/3(control), Subsystem C_Y_A/3(control)
  phi_t/1 -> Subsystem C_Z_A/4(phi_t), Subsystem C_Y_A/4(phi_t)

== system Missile_Aerodynamics/UAS Model/Forces1/Total Force & Moment/Gravity ==
  cE_B : Inport
  Constant : Constant  Value=0
  Constant1 : Constant  Value=Mass
  Display : Display
  Display1 : Display
  "Gravity vector in body frame " : Product  Multiplication=Matrix(*)  SaturateOnIntegerOverflow=on  InputSameDT=on  OutDataTypeStr=Inherit: Same as first input
  Mux1 : Mux  Inputs=3
  g : Gain  Gain=UNIT_GRAV
  Gravity : Outport
  wires:
  Constant1/1 -> g/1
  "Gravity vector in body frame "/1 -> Display/1, Gravity/1
  g/1 -> Mux1/3
  Mux1/1 -> "Gravity vector in body frame "/2
  cE_B/1 -> Display1/1, "Gravity vector in body frame "/1
  Constant/1 -> Mux1/1, Mux1/2

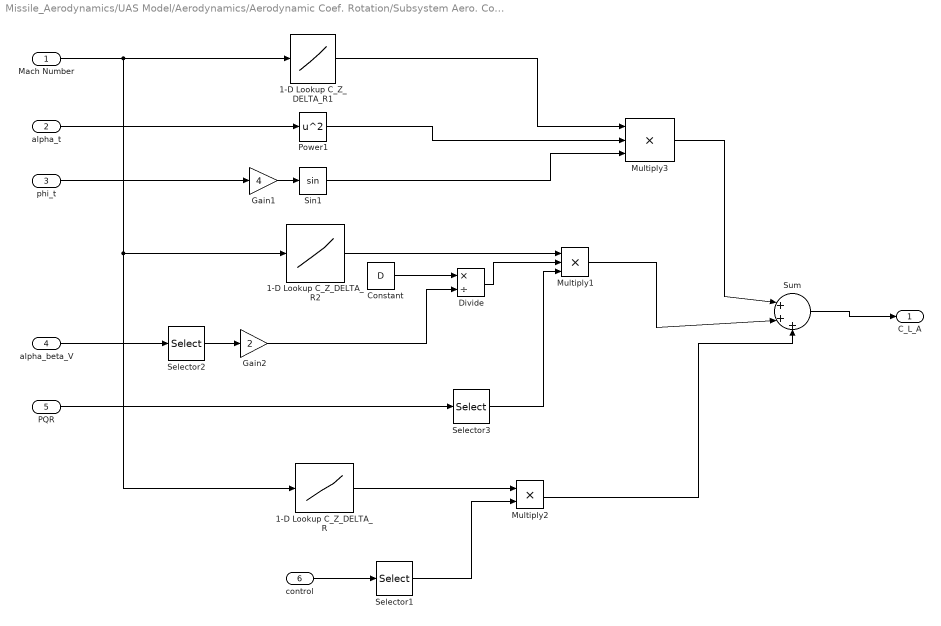
== system Missile_Aerodynamics/UAS Model/Aerodynamics/Aerodynamic Coef. Rotation/Subsystem Aero. Coef. Rotation/Subsystem C_L_A  ==
  Mach Number : Inport
  alpha_t : Inport  Port=2
  phi_t : Inport  Port=3
  alpha_beta_V : Inport  Port=4
  PQR : Inport  Port=5
  control : Inport  Port=6
  1-D Lookup C_Z_DELTA_R : Lookup_n-D  NumberOfTableDimensions=1  BreakpointsForDimension1=Tbl_MACH  Table=Tbl_CL_DEL_R  InternalRulePriority=Speed  RndMeth=Simplest  InputSameDT=on
  1-D Lookup C_Z_DELTA_R1 : Lookup_n-D  NumberOfTableDimensions=1  BreakpointsForDimension1=Tbl_MACH  Table=Tbl_CL_ALPHAT  InternalRulePriority=Speed  RndMeth=Simplest  InputSameDT=on
  1-D Lookup C_Z_DELTA_R2 : Lookup_n-D  NumberOfTableDimensions=1  BreakpointsForDimension1=Tbl_MACH  Table=Tbl_CL_P  InternalRulePriority=Speed  RndMeth=Simplest  InputSameDT=on
  Constant : Constant  Value=D
  Divide : Product  Inputs=*/
  Gain1 : Gain  Gain=4
  Gain2 : Gain  Gain=2
  Multiply1 : Product  Inputs=3
  Multiply2 : Product
  Multiply3 : Product  Inputs=3
  Power1 : Math  Operator=square  SaturateOnIntegerOverflow=on
  Selector1 : Selector  InputPortWidth=3  IndexOptions=Index vector (dialog)  Indices=[1]  OutputSizes=1
  Selector2 : Selector  InputPortWidth=3  IndexOptions=Index vector (dialog)  Indices=[3]  OutputSizes=1
  Selector3 : Selector  InputPortWidth=3  IndexOptions=Index vector (dialog)  Indices=[1]  OutputSizes=1
  Sin1 : Trigonometry
  Sum : Sum  Inputs=|+++
  C_L_A : Outport
  wires:
  1-D Lookup C_Z_DELTA_R1/1 -> Multiply3/1
  alpha_t/1 -> Power1/1
  Sum/1 -> C_L_A/1
  Mach Number/1 -> 1-D Lookup C_Z_DELTA_R/1, 1-D Lookup C_Z_DELTA_R2/1, 1-D Lookup C_Z_DELTA_R1/1
  1-D Lookup C_Z_DELTA_R2/1 -> Multiply1/1
  1-D Lookup C_Z_DELTA_R/1 -> Multiply2/1
  Multiply2/1 -> Sum/3
  Power1/1 -> Multiply3/2
  Sin1/1 -> Multiply3/3
  phi_t/1 -> Gain1/1
  Gain1/1 -> Sin1/1
  alpha_beta_V/1 -> Selector2/1
  Multiply3/1 -> Sum/1
  Multiply1/1 -> Sum/2
  Constant/1 -> Divide/1
  Selector2/1 -> Gain2/1
  Gain2/1 -> Divide/2
  Divide/1 -> Multiply1/2
  PQR/1 -> Selector3/1
  Selector3/1 -> Multiply1/3
  control/1 -> Selector1/1
  Selector1/1 -> Multiply2/2

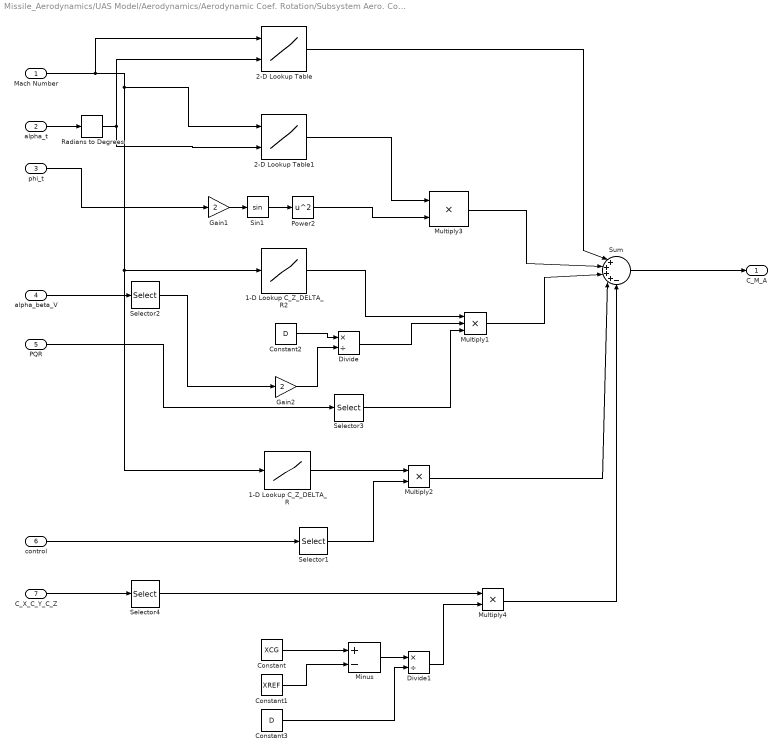
== system Missile_Aerodynamics/UAS Model/Aerodynamics/Aerodynamic Coef. Rotation/Subsystem Aero. Coef. Rotation/Subsystem C_M_A  ==
  Mach Number : Inport
  alpha_t : Inport  Port=2
  phi_t : Inport  Port=3
  alpha_beta_V : Inport  Port=4
  PQR : Inport  Port=5
  control : Inport  Port=6
  C_X_C_Y_C_Z : Inport  Port=7
  1-D Lookup C_Z_DELTA_R : Lookup_n-D  NumberOfTableDimensions=1  BreakpointsForDimension1=Tbl_MACH  Table=Tbl_CM_DEL_P  InternalRulePriority=Speed  RndMeth=Simplest  InputSameDT=on
  1-D Lookup C_Z_DELTA_R2 : Lookup_n-D  NumberOfTableDimensions=1  BreakpointsForDimension1=Tbl_MACH  Table=Tbl_CM_Q  DiagnosticForOutOfRangeInput=Warning  InternalRulePriority=Speed  RndMeth=Simplest  InputSameDT=on
  2-D Lookup Table : Lookup_n-D  BreakpointsForDimension1=Tbl_MACH  BreakpointsForDimension2=Tbl_ALPHAT  Table=Tbl_CM_0  DiagnosticForOutOfRangeInput=Warning  InternalRulePriority=Speed  RndMeth=Simplest  InputSameDT=on
  2-D Lookup Table1 : Lookup_n-D  BreakpointsForDimension1=Tbl_MACH  BreakpointsForDimension2=Tbl_ALPHAT  Table=Tbl_CM_PHIT  InternalRulePriority=Speed  RndMeth=Simplest  InputSameDT=on
  Constant : Constant  Value=XCG
  Constant1 : Constant  Value=XREF
  Constant2 : Constant  Value=D
  Constant3 : Constant  Value=D
  Divide : Product  Inputs=*/
  Divide1 : Product  Inputs=*/
  Gain1 : Gain  Gain=2
  Gain2 : Gain  Gain=2
  Minus : Sum  Inputs=+-
  Multiply1 : Product  Inputs=3
  Multiply2 : Product
  Multiply3 : Product
  Multiply4 : Product
  Power2 : Math  Operator=square  SaturateOnIntegerOverflow=on
  Radians to Degrees : simulink_extras/Transformations/Radians to Degrees
  Selector1 : Selector  InputPortWidth=3  IndexOptions=Index vector (dialog)  Indices=[2]  OutputSizes=1
  Selector2 : Selector  InputPortWidth=3  IndexOptions=Index vector (dialog)  Indices=[3]  OutputSizes=1
  Selector3 : Selector  InputPortWidth=3  IndexOptions=Index vector (dialog)  Indices=[2]  OutputSizes=1
  Selector4 : Selector  InputPortWidth=3  IndexOptions=Index vector (dialog)  Indices=[3]  OutputSizes=1
  Sin1 : Trigonometry
  Sum : Sum  Inputs=|++++-
  C_M_A : Outport
  wires:
  2-D Lookup Table/1 -> Sum/1
  Mach Number/1 -> 2-D Lookup Table/1, 2-D Lookup Table1/1, 1-D Lookup C_Z_DELTA_R/1, 1-D Lookup C_Z_DELTA_R2/1
  1-D Lookup C_Z_DELTA_R2/1 -> Multiply1/1
  1-D Lookup C_Z_DELTA_R/1 -> Multiply2/1
  Multiply2/1 -> Sum/4
  Sin1/1 -> Power2/1
  phi_t/1 -> Gain1/1
  Gain1/1 -> Sin1/1
  alpha_beta_V/1 -> Selector2/1
  Selector2/1 -> Gain2/1
  Gain2/1 -> Divide/2
  Divide/1 -> Multiply1/2
  PQR/1 -> Selector3/1
  Selector3/1 -> Multiply1/3
  control/1 -> Selector1/1
  Selector1/1 -> Multiply2/2
  2-D Lookup Table1/1 -> Multiply3/1
  Power2/1 -> Multiply3/2
  C_X_C_Y_C_Z/1 -> Selector4/1
  Constant/1 -> Minus/1
  Constant1/1 -> Minus/2
  Constant2/1 -> Divide/1
  Minus/1 -> Divide1/1
  Constant3/1 -> Divide1/2
  Selector4/1 -> Multiply4/1
  Divide1/1 -> Multiply4/2
  Multiply4/1 -> Sum/5
  Multiply1/1 -> Sum/3
  Multiply3/1 -> Sum/2
  alpha_t/1 -> Radians to Degrees/1
  Radians to Degrees/1 -> 2-D Lookup Table1/2, 2-D Lookup Table/2
  Sum/1 -> C_M_A/1

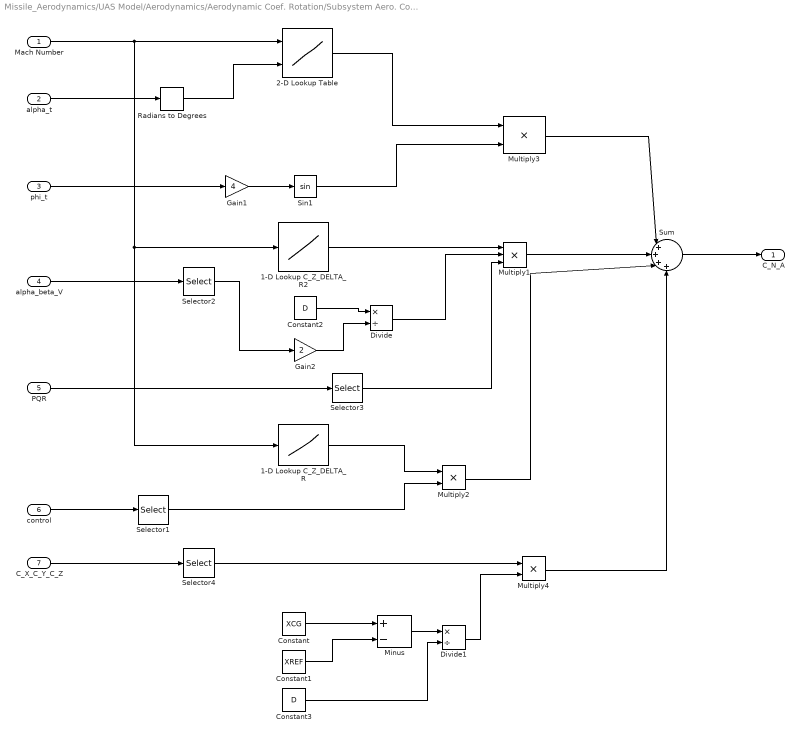
== system Missile_Aerodynamics/UAS Model/Aerodynamics/Aerodynamic Coef. Rotation/Subsystem Aero. Coef. Rotation/Subsystem C_N_A ==
  Mach Number : Inport
  alpha_t : Inport  Port=2
  phi_t : Inport  Port=3
  alpha_beta_V : Inport  Port=4
  PQR : Inport  Port=5
  control : Inport  Port=6
  C_X_C_Y_C_Z : Inport  Port=7
  1-D Lookup C_Z_DELTA_R : Lookup_n-D  NumberOfTableDimensions=1  BreakpointsForDimension1=Tbl_MACH  Table=Tbl_CN_DEL_Y  InternalRulePriority=Speed  RndMeth=Simplest  InputSameDT=on
  1-D Lookup C_Z_DELTA_R2 : Lookup_n-D  NumberOfTableDimensions=1  BreakpointsForDimension1=Tbl_MACH  Table=Tbl_CN_R  InternalRulePriority=Speed  RndMeth=Simplest  InputSameDT=on
  2-D Lookup Table : Lookup_n-D  BreakpointsForDimension1=Tbl_MACH  BreakpointsForDimension2=Tbl_ALPHAT  Table=Tbl_CN_PHIT  InternalRulePriority=Speed  RndMeth=Simplest  InputSameDT=on
  Constant : Constant  Value=XCG
  Constant1 : Constant  Value=XREF
  Constant2 : Constant  Value=D
  Constant3 : Constant  Value=D
  Divide : Product  Inputs=*/
  Divide1 : Product  Inputs=*/
  Gain1 : Gain  Gain=4
  Gain2 : Gain  Gain=2
  Minus : Sum  Inputs=+-
  Multiply1 : Product  Inputs=3
  Multiply2 : Product
  Multiply3 : Product
  Multiply4 : Product
  Radians to Degrees : simulink_extras/Transformations/Radians to Degrees
  Selector1 : Selector  InputPortWidth=3  IndexOptions=Index vector (dialog)  Indices=[3]  OutputSizes=1
  Selector2 : Selector  InputPortWidth=3  IndexOptions=Index vector (dialog)  Indices=[3]  OutputSizes=1
  Selector3 : Selector  InputPortWidth=3  IndexOptions=Index vector (dialog)  Indices=[3]  OutputSizes=1
  Selector4 : Selector  InputPortWidth=3  IndexOptions=Index vector (dialog)  Indices=[2]  OutputSizes=1
  Sin1 : Trigonometry
  Sum : Sum  Inputs=|++++
  C_N_A : Outport
  wires:
  2-D Lookup Table/1 -> Multiply3/1
  alpha_t/1 -> Radians to Degrees/1
  Sum/1 -> C_N_A/1
  Mach Number/1 -> 2-D Lookup Table/1, 1-D Lookup C_Z_DELTA_R/1, 1-D Lookup C_Z_DELTA_R2/1
  1-D Lookup C_Z_DELTA_R2/1 -> Multiply1/1
  1-D Lookup C_Z_DELTA_R/1 -> Multiply2/1
  Multiply2/1 -> Sum/3
  Sin1/1 -> Multiply3/2
  phi_t/1 -> Gain1/1
  Gain1/1 -> Sin1/1
  alpha_beta_V/1 -> Selector2/1
  Selector2/1 -> Gain2/1
  Divide/1 -> Multiply1/2
  PQR/1 -> Selector3/1
  Selector3/1 -> Multiply1/3
  control/1 -> Selector1/1
  Selector1/1 -> Multiply2/2
  C_X_C_Y_C_Z/1 -> Selector4/1
  Constant/1 -> Minus/1
  Constant1/1 -> Minus/2
  Constant2/1 -> Divide/1
  Minus/1 -> Divide1/1
  Constant3/1 -> Divide1/2
  Selector4/1 -> Multiply4/1
  Divide1/1 -> Multiply4/2
  Multiply4/1 -> Sum/4
  Multiply1/1 -> Sum/2
  Multiply3/1 -> Sum/1
  Radians to Degrees/1 -> 2-D Lookup Table/2
  Gain2/1 -> Divide/2

== system Missile_Aerodynamics/UAS Model/Aerodynamics/Aerodynamic Coef. Translation/Subsystem Aero. Coef. Translation/Subsystem C_X_A ==
  Mach Number : Inport
  alpha_t : Inport  Port=2
  delta_eff : Inport  Port=3
  1-D Lookup C_X_0 : Lookup_n-D  NumberOfTableDimensions=1  BreakpointsForDimension1=Tbl_MACH  Table=Tbl_CX_0  DiagnosticForOutOfRangeInput=Error  InternalRulePriority=Speed  RndMeth=Simplest  InputSameDT=on
  1-D Lookup C_X_ALPHA_T : Lookup_n-D  NumberOfTableDimensions=1  BreakpointsForDimension1=Tbl_MACH  BeginIndexSearchUsingPreviousIndexResult=on  Table=Tbl_CX_ALPHAT  DiagnosticForOutOfRangeInput=Error  InternalRulePriority=Speed  RndMeth=Simplest  InputSameDT=on
  1-D Lookup C_X_DELTA_EFF : Lookup_n-D  NumberOfTableDimensions=1  BreakpointsForDimension1=Tbl_MACH  Table=Tbl_CX_DEL_EFF  DiagnosticForOutOfRangeInput=Error  InternalRulePriority=Speed  RndMeth=Simplest  InputSameDT=on
  Display : Display
  Multiply : Product
  Multiply1 : Product
  Scope : Scope
  Square : Math  Operator=square  SaturateOnIntegerOverflow=on
  Sum : Sum  Inputs=|+++
  C_X_A : Outport
  wires:
  Multiply/1 -> Sum/2
  Multiply1/1 -> Display/1, Sum/3
  1-D Lookup C_X_DELTA_EFF/1 -> Multiply1/1
  1-D Lookup C_X_ALPHA_T/1 -> Multiply/1
  1-D Lookup C_X_0/1 -> Sum/1
  Mach Number/1 -> 1-D Lookup C_X_DELTA_EFF/1, 1-D Lookup C_X_ALPHA_T/1, Scope/1, 1-D Lookup C_X_0/1
  Sum/1 -> C_X_A/1
  alpha_t/1 -> Multiply/2
  delta_eff/1 -> Square/1
  Square/1 -> Multiply1/2

== system Missile_Aerodynamics/UAS Model/Aerodynamics/Aerodynamic Coef. Translation/Subsystem Aero. Coef. Translation/Subsystem C_Y_A ==
  Mach Number : Inport
  alpha_t : Inport  Port=2
  control : Inport  Port=3
  phi_t : Inport  Port=4
  1-D Lookup C_Y_DELTA_Y : Lookup_n-D  NumberOfTableDimensions=1  BreakpointsForDimension1=Tbl_MACH  Table=Tbl_CY_DEL_Y  InternalRulePriority=Speed  RndMeth=Simplest  InputSameDT=on
  2-D Lookup CY_PHIT : Lookup_n-D  BreakpointsForDimension1=Tbl_MACH  BreakpointsForDimension2=Tbl_ALPHAT  Table=Tbl_CY_PHIT  InternalRulePriority=Speed  RndMeth=Simplest  InputSameDT=on
  Gain : Gain  Gain=4
  Multiply1 : Product
  Multiply2 : Product
  Radians to Degrees : simulink_extras/Transformations/Radians to Degrees
  Sin : Trigonometry
  Sum : Sum  Inputs=|++
  delta_y : Selector  InputPortWidth=3  IndexOptions=Index vector (dialog)  Indices=[3]  OutputSizes=1
  C_Y_A : Outport
  wires:
  Multiply1/1 -> Sum/2
  1-D Lookup C_Y_DELTA_Y/1 -> Multiply1/1
  2-D Lookup CY_PHIT/1 -> Multiply2/1
  Mach Number/1 -> 1-D Lookup C_Y_DELTA_Y/1, 2-D Lookup CY_PHIT/1
  Sum/1 -> C_Y_A/1
  Gain/1 -> Sin/1
  phi_t/1 -> Gain/1
  control/1 -> delta_y/1
  alpha_t/1 -> Radians to Degrees/1
  delta_y/1 -> Multiply1/2
  Sin/1 -> Multiply2/2
  Multiply2/1 -> Sum/1
  Radians to Degrees/1 -> 2-D Lookup CY_PHIT/2

== system Missile_Aerodynamics/UAS Model/Aerodynamics/Aerodynamic Coef. Translation/Subsystem Aero. Coef. Translation/Subsystem C_Z_A ==
  Mach Number : Inport
  alpha_t : Inport  Port=2
  control : Inport  Port=3
  phi_t : Inport  Port=4
  1-D Lookup C_Z_DELTA_P : Lookup_n-D  NumberOfTableDimensions=1  BreakpointsForDimension1=Tbl_MACH  Table=Tbl_CZ_DEL_P  InternalRulePriority=Speed  RndMeth=Simplest  InputSameDT=on
  2-D Lookup C_Z_0 : Lookup_n-D  BreakpointsForDimension1=Tbl_MACH  BreakpointsForDimension2=Tbl_ALPHAT  Table=Tbl_CZ_0  DiagnosticForOutOfRangeInput=Warning  InternalRulePriority=Speed  RndMeth=Simplest  InputSameDT=on
  2-D Lookup C_Z_PHI_T : Lookup_n-D  BreakpointsForDimension1=Tbl_MACH  BreakpointsForDimension2=Tbl_ALPHAT  Table=Tbl_CZ_PHIT  InternalRulePriority=Speed  RndMeth=Simplest  InputSameDT=on
  Gain : Gain  Gain=2
  Multiply1 : Product
  Multiply2 : Product
  Power : Math  Operator=square  SaturateOnIntegerOverflow=on
  Radians to Degrees : simulink_extras/Transformations/Radians to Degrees
  Sin : Trigonometry
  Sum : Sum  Inputs=|+++
  delta_p : Selector  InputPortWidth=3  IndexOptions=Index vector (dialog)  Indices=[2]  OutputSizes=1
  C_Z_A : Outport
  wires:
  2-D Lookup C_Z_0/1 -> Sum/1
  delta_p/1 -> Multiply2/2
  alpha_t/1 -> Radians to Degrees/1
  control/1 -> delta_p/1
  Sum/1 -> C_Z_A/1
  Mach Number/1 -> 2-D Lookup C_Z_PHI_T/1, 1-D Lookup C_Z_DELTA_P/1, 2-D Lookup C_Z_0/1
  2-D Lookup C_Z_PHI_T/1 -> Multiply1/1
  Multiply1/1 -> Sum/2
  Gain/1 -> Sin/1
  phi_t/1 -> Gain/1
  Sin/1 -> Power/1
  Power/1 -> Multiply1/2
  1-D Lookup C_Z_DELTA_P/1 -> Multiply2/1
  Multiply2/1 -> Sum/3
  Radians to Degrees/1 -> 2-D Lookup C_Z_0/2, 2-D Lookup C_Z_PHI_T/2
